simulink model "detect_cornor_1"  (R2016a)
settings: Solver=VariableStepAuto  StartTime=0.0  StopTime=1  RelTol=1e-3
undefined symbols (not defined in the file): fspecial, Rec, SDTV
libraries: visionconversions x4, simulink x1, visionanalysis x1, visiontextngfix x1, visionsources x1
settings Model: Creator=Yewly  LastModifiedBy=Yewly
settings GRTTargetCC: GeneratePreprocessorConditionals=Use local settings

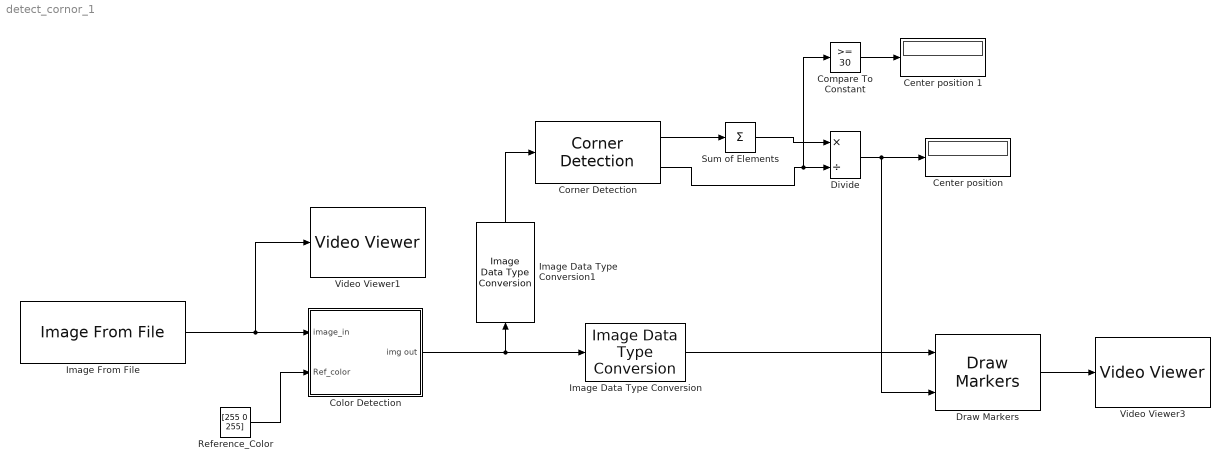
== system detect_cornor_1 ==
  "Center position " : Display
      settings: Decimation=100
  Center position 1 : Display
      settings: Decimation=100
  Color Detection : Subsystem
  Compare To Constant : simulink/Logic and Bit Operations/Compare To Constant  relop=>=  const=30  OutDataTypeStr=boolean
  Corner Detection : visionanalysis/Corner Detection  method=Harris corner detection (Harris & Stephens)  factor=0.04  filter=fspecial('gaussian', [1 5], 1.5)  thrInten=0.1  thrAngle=157.5  output=Obsolete9b  outputInUse=Corner location  maxNum=1000  thrMetric=0.005  neighborSize=[13 13]  isOutVarDim=off  accumMode=Binary point scaling  accumWordLength=32  accumFracLength=0  prodOutputMode=Binary point scaling  prodOutputWordLength=32  prodOutputFracLength=0  memoryMode=Binary point scaling  memoryWordLength=32  memoryFracLength=0  firstCoeffMode=Specify word length  firstCoeffWordLength=16  firstCoeffFracLength=16  roundingMode=Floor  overflowMode=off
  Divide : Product  Inputs=*/
  Draw Markers : visiontextngfix/Draw Markers  shape=Circle  size=3  fill=off  fillClrSource=Specify via dialog  display=Black  intensity=200  color=1  opacity=0.6  viewport=Entire image  antialiasing=off  inType=Obsolete  imagePorts=One multidimensional signal  prodOutputMode=Binary point scaling  prodOutputWordLength=32  prodOutputFracLength=14  memoryMode=Specify word length  memoryWordLength=16  memoryFracLength=14  roundingMode=Floor  overflowMode=off
  Image Data Type Conversion : visionconversions/Image Data Type Conversion  outDT=double  isSigned=on  wordLen=16  numFracBits=0
  Image Data Type Conversion1 : visionconversions/Image Data Type Conversion  outDT=double  isSigned=on  wordLen=16  numFracBits=0
  Image From File : visionsources/Image From File  Tag=vipblks_nd  FileName=color6.jpg  imagePorts=One multidimensional signal  Ts=1  ImageDataType=double  Signed=on  WordLength=16  sdImageDataType=uint(8)  FractionLengthMode=User-defined  FractionLength=15  OutPortLabels=R|G|B
  Reference_Color : Constant  Value=[255 0 255]  OutDataTypeStr=uint8
  Sum of Elements : Sum  Inputs=+  CollapseMode=Specified dimension
  Video Viewer1 : VideoViewer  FigPos=[208.2 742 540 585.6]
  Video Viewer3 : VideoViewer  FigPos=[641 738.8 540 585.6]
  wires:
  Reference_Color/1 -> Color Detection/2(Ref_color)
  Color Detection/1(img out) -> Image Data Type Conversion1/1, Image Data Type Conversion/1
  Corner Detection/1 -> Sum of Elements/1
  Corner Detection/2 -> Compare To Constant/1, Divide/2
  Image Data Type Conversion1/1 -> Corner Detection/1
  Divide/1 -> "Center position "/1, Draw Markers/2
  Image From File/1 -> Video Viewer1/1, Color Detection/1("image_in ")
  Draw Markers/1 -> Video Viewer3/1
  Image Data Type Conversion/1 -> Draw Markers/1
  Sum of Elements/1 -> Divide/1
  Compare To Constant/1 -> Center position 1/1

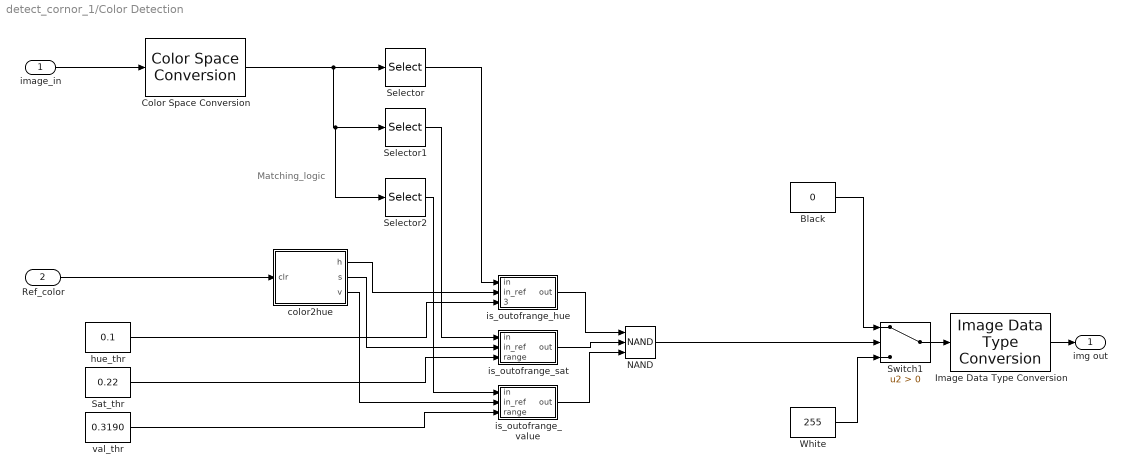
== system detect_cornor_1/Color Detection ==
  note: Matching_logic
  "image_in " : Inport
  Ref_color : Inport  Port=2
  Black : Constant  Value=0
  Color Space Conversion : visionconversions/Color Space  Conversion  conversion=Obsolete  conversionActive=R'G'B' to HSV  wp_str=D65  rec=Rec. 601 (SDTV)  sys=1125/60/2:1  imagePorts=One multidimensional signal
  Image Data Type Conversion : visionconversions/Image Data Type Conversion  outDT=boolean  isSigned=on  wordLen=16  numFracBits=0
  NAND : Logic  Operator=NAND  Inputs=3  IconShape=distinctive  AllPortsSameDT=off  OutDataTypeStr=boolean
  Sat_thr : Constant  Value=0.22
  Selector : Selector  NumberOfDimensions=3  InputPortWidth=3  IndexOptions=Select all,Select all,Index vector (dialog)  Indices=1,1,1  OutputSizes=1,1,1
  Selector1 : Selector  NumberOfDimensions=3  InputPortWidth=3  IndexOptions=Select all,Select all,Index vector (dialog)  Indices=1,1,2  OutputSizes=1,1,1
  Selector2 : Selector  NumberOfDimensions=3  InputPortWidth=3  IndexOptions=Select all,Select all,Index vector (dialog)  Indices=1,1,3  OutputSizes=1,1,1
  Switch1 : Switch  Criteria=u2 > Threshold  OutDataTypeStr=uint8
  White : Constant  Value=255
  color2hue : MATLAB Function  TreatAsAtomicUnit=on
  hue_thr : Constant  Value=0.1
  is_outofrange_hue : Subsystem
  "is_outofrange_sat " : Subsystem
  is_outofrange_value : Subsystem
  val_thr : Constant  Value=0.3190
  img out : Outport
  wires:
  hue_thr/1 -> is_outofrange_hue/3("threshold ")
  is_outofrange_value/1(out) -> NAND/3
  is_outofrange_hue/1(out) -> NAND/1
  Sat_thr/1 -> "is_outofrange_sat "/3("range ")
  val_thr/1 -> is_outofrange_value/3("range ")
  Selector2/1 -> is_outofrange_value/1(in)
  color2hue/3(v) -> is_outofrange_value/2(in_ref)
  color2hue/1(h) -> is_outofrange_hue/2(in_ref)
  Selector/1 -> is_outofrange_hue/1(in)
  Ref_color/1 -> color2hue/1(clr)
  "is_outofrange_sat "/1(out) -> NAND/2
  color2hue/2(s) -> "is_outofrange_sat "/2(in_ref)
  Selector1/1 -> "is_outofrange_sat "/1(in)
  Switch1/1 -> Image Data Type Conversion/1
  NAND/1 -> Switch1/2
  Black/1 -> Switch1/1
  "image_in "/1 -> Color Space Conversion/1
  Color Space Conversion/1 -> Selector2/1, Selector1/1, Selector/1
  Image Data Type Conversion/1 -> img out/1
  White/1 -> Switch1/3

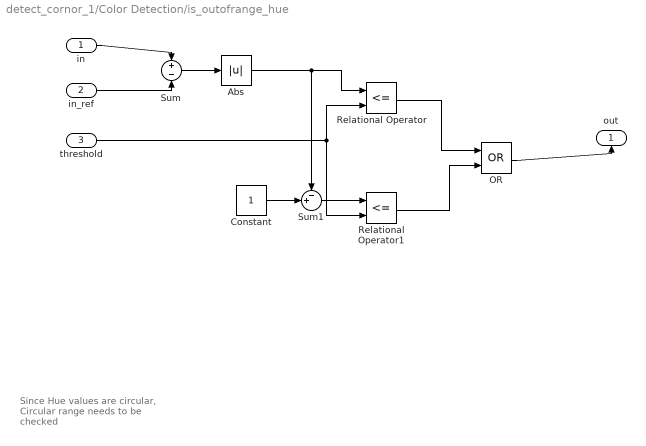
== system detect_cornor_1/Color Detection/is_outofrange_hue ==
  note: Since Hue values are circular, Circular range needs to be checked
  in : Inport
  in_ref : Inport  Port=2
  "threshold " : Inport  Port=3
  Abs : Abs
  Constant : Constant
  "OR " : Logic  Operator=OR  AllPortsSameDT=off  OutDataTypeStr=boolean
  Relational Operator : RelationalOperator  Operator=<=  OutDataTypeStr=boolean
  Relational Operator1 : RelationalOperator  Operator=<=  OutDataTypeStr=boolean
  Sum : Sum  Inputs=+|-
  Sum1 : Sum  Inputs=-+|
  out : Outport
  wires:
  in/1 -> Sum/1
  in_ref/1 -> Sum/2
  Sum/1 -> Abs/1
  Abs/1 -> Sum1/1, Relational Operator/1
  "threshold "/1 -> Relational Operator1/2, Relational Operator/2
  Constant/1 -> Sum1/2
  Sum1/1 -> Relational Operator1/1
  Relational Operator/1 -> "OR "/1
  Relational Operator1/1 -> "OR "/2
  "OR "/1 -> out/1

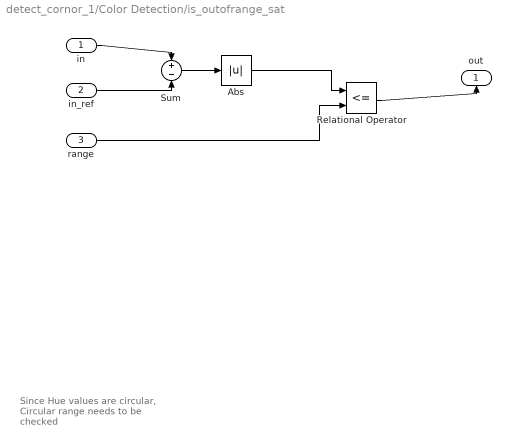
== system detect_cornor_1/Color Detection/is_outofrange_sat  ==
  note: Since Hue values are circular, Circular range needs to be checked
  in : Inport
  in_ref : Inport  Port=2
  "range " : Inport  Port=3
  Abs : Abs
  Relational Operator : RelationalOperator  Operator=<=  OutDataTypeStr=boolean
  Sum : Sum  Inputs=+|-
  out : Outport
  wires:
  in/1 -> Sum/1
  in_ref/1 -> Sum/2
  Sum/1 -> Abs/1
  Abs/1 -> Relational Operator/1
  "range "/1 -> Relational Operator/2
  Relational Operator/1 -> out/1

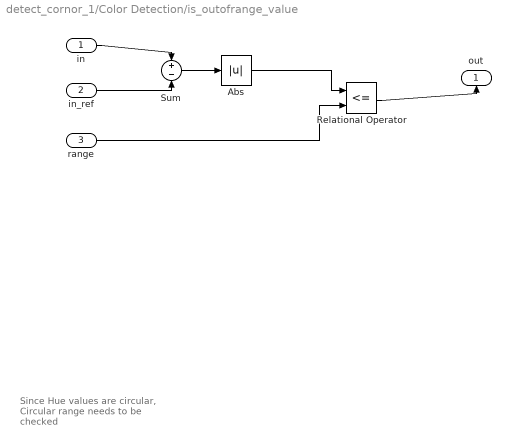
== system detect_cornor_1/Color Detection/is_outofrange_value ==
  note: Since Hue values are circular, Circular range needs to be checked
  in : Inport
  in_ref : Inport  Port=2
  "range " : Inport  Port=3
  Abs : Abs
  Relational Operator : RelationalOperator  Operator=<=  OutDataTypeStr=boolean
  Sum : Sum  Inputs=+|-
  out : Outport
  wires:
  in/1 -> Sum/1
  in_ref/1 -> Sum/2
  Sum/1 -> Abs/1
  Abs/1 -> Relational Operator/1
  "range "/1 -> Relational Operator/2
  Relational Operator/1 -> out/1

== matlab function detect_cornor_1/Color Detection/color2hue ==
  data: clr input; h output; s output; v output
function [h,s,v] = color2hue(clr)
%#codegen

hsv = rgb2hsv(double(clr')/255.0);
h = hsv(1);
s = hsv(2);
v = hsv(3);
